simulink model "laba_3"  (Simulink 9.2)
settings: Solver=FixedStepAuto  StartTime=0.0  StopTime=10  FixedStep=0.0001  RelTol=1e-3  EnableMultiTasking=on
settings Model: Creator=student  LastModifiedBy=murad  SnapshotInterval=100
settings OptimizationCC: ExpressionDepthLimit=2147483647
settings DebuggingCC: SolverPrmCheckMsg=warning

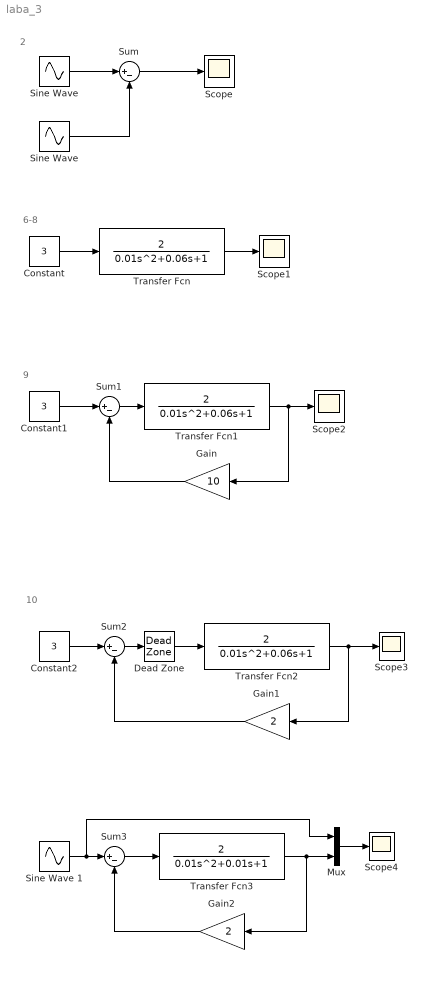
== system laba_3 ==
  note: 10
  note: 6-8
  note: 2
  note: 9
  Constant : Constant  Value=3
  Constant1 : Constant  Value=3
  Constant2 : Constant  Value=3
  Dead Zone : DeadZone  LowerValue=1  UpperValue=1.5  SaturateOnIntegerOverflow=on
  Gain : Gain  Gain=10
  Gain1 : Gain  Gain=2
  Gain2 : Gain  Gain=2
  Mux : Mux  Inputs=2
  Scope{,1..4} (5 alike) : Scope
  Sine Wave : Sin  Amplitude=3  Frequency=5  SampleTime=0
  "Sine Wave " : Sin  Amplitude=2  Frequency=2  SampleTime=0
  Sine Wave 1 : Sin  Amplitude=2.7  Frequency=22  SampleTime=0
  Sum{,1..3} (4 alike) : Sum  Inputs=|+-
  Transfer Fcn : TransferFcn  Numerator=[2]  Denominator=[0.01 0.06 1]
  Transfer Fcn1 : TransferFcn  Numerator=[2]  Denominator=[0.01 0.06 1]
  Transfer Fcn2 : TransferFcn  Numerator=[2]  Denominator=[0.01 0.06 1]
  Transfer Fcn3 : TransferFcn  Numerator=[2]  Denominator=[0.01 0.01 1]
  wires:
  Sum/1 -> Scope/1
  "Sine Wave "/1 -> Sum/1
  Sine Wave/1 -> Sum/2
  Constant/1 -> Transfer Fcn/1
  Transfer Fcn/1 -> Scope1/1
  Transfer Fcn1/1 -> Scope2/1, Gain/1
  Sum1/1 -> Transfer Fcn1/1
  Constant1/1 -> Sum1/1
  Gain/1 -> Sum1/2
  Transfer Fcn2/1 -> Scope3/1, Gain1/1
  Gain1/1 -> Sum2/2
  Constant2/1 -> Sum2/1
  Sum2/1 -> Dead Zone/1
  Dead Zone/1 -> Transfer Fcn2/1
  Sine Wave 1/1 -> Mux/1, Sum3/1
  Sum3/1 -> Transfer Fcn3/1
  Gain2/1 -> Sum3/2
  Mux/1 -> Scope4/1
  Transfer Fcn3/1 -> Gain2/1, Mux/2
